simulink model "simu1"  (R2022a)
settings: Solver=VariableStepAuto  StartTime=0.0  StopTime=20.0  RelTol=1e-3
values from neighbouring files (symbols this model uses):
  x0 = 0    [lista08.m]
settings Model: Creator=marcone.faria  LastModifiedBy=marcone.faria
settings DataIOCC: SaveFormat=Array  ReturnWorkspaceOutputs=off

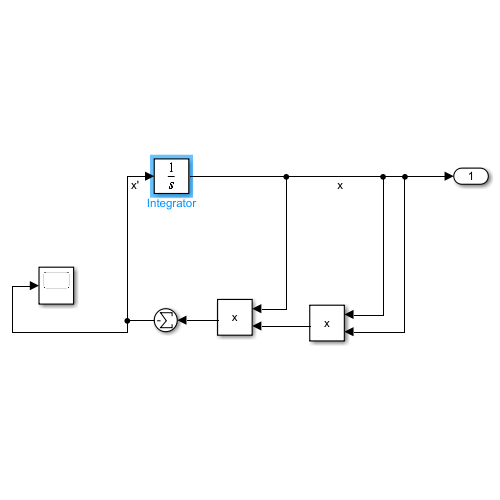
[thumbnail: Simulink's stored preview of the top-level diagram]
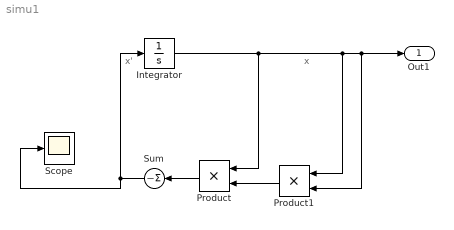
== system simu1 ==
  note: x
  note: x'
  Integrator : Integrator  InitialCondition=x0
  Product : Product
  Product1 : Product
  Scope : Scope
  Sum : Sum  Inputs=-
  Out1 : Outport
  wires:
  Sum/1 -> Integrator/1, Scope/1
  Product/1 -> Sum/1
  Integrator/1 -> Product1/2, Out1/1, Product1/1, Product/1
  Product1/1 -> Product/2
